simulink model "regulador_apenas"  (R2016a)
settings: Solver=VariableStepAuto  StartTime=0.0  StopTime=10.0  RelTol=1e-3
values from neighbouring files (symbols this model uses):
  AA = A    [identify_v2.m]    (also in statespace.mat = [5.5279791139 1 0 0 0 0 0 -13.5203927489 0 1 0 0 ... (49 ele)
  BB = B    [identify_v2.m]    (also in statespace.mat = [1 0 0 0 0 0 0])
  CC = C    [identify_v2.m]    (also in statespace.mat = [-3.36334453848e-05 3.71652773519e-05 -0.000281908447517 0.0)
  Nbar = Nu+K*Nx    [controller.m]
  Ts = mean(diff(ts))    [controller.m]    (also in identify.m; identify_v2.m; simubarra1.m = 0.01)
undefined symbols (not defined in the file or in its folder): K
settings Model: Creator=Mihir  LastModifiedBy=Mihir

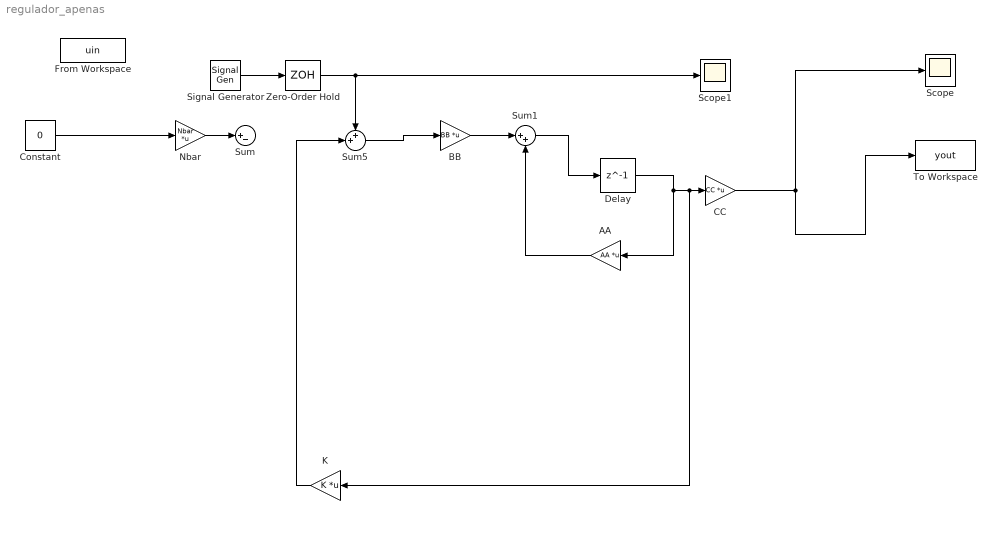
== system regulador_apenas ==
  AA : Gain  Gain=AA  Multiplication=Matrix(K*u)
  BB : Gain  Gain=BB  Multiplication=Matrix(K*u)
  CC : Gain  Gain=CC  Multiplication=Matrix(K*u)
  Constant : Constant  Value=0  SampleTime=Ts
  Delay : Delay  DelayLength=1  InitialCondition=0
  From Workspace : FromWorkspace  VariableName=uin  SampleTime=Ts
  K : Gain  Gain=K  Multiplication=Matrix(K*u)
  Nbar : Gain  Gain=Nbar  Multiplication=Matrix(K*u)
  Scope : Scope
  Scope1 : Scope
  Signal Generator : SignalGenerator  WaveForm=square  Frequency=0.1  Units=rad/sec
  Sum : Sum  Inputs=|+-
  Sum1 : Sum  Inputs=|++
  Sum5 : Sum  Inputs=++|
  To Workspace : ToWorkspace  VariableName=yout  SaveFormat=Structure With Time  SampleTime=-1
  Zero-Order Hold : ZeroOrderHold  SampleTime=Ts
  wires:
  AA/1 -> Sum1/2
  Delay/1 -> K/1, CC/1, AA/1
  CC/1 -> To Workspace/1, Scope/1
  Sum1/1 -> Delay/1
  BB/1 -> Sum1/1
  Nbar/1 -> Sum/1
  Signal Generator/1 -> Zero-Order Hold/1
  Zero-Order Hold/1 -> Sum5/1, Scope1/1
  Sum5/1 -> BB/1
  Constant/1 -> Nbar/1
  K/1 -> Sum5/2
